simulink model "power_microgrid_v3_analytic"  (R2018b)
settings: Solver=ode23tb  StartTime=0.0  StopTime=24*60*60  FixedStep=1/(1000)  MaxStep=60  RelTol=1e-4
PreLoadFcn:
  | load('solar_load_data_24h.mat')
PostLoadFcn:
  | data = xlsread('Domestic_data_all_x3','Sheet1');
  | breakpoints1 = data(2:end,1)'
  | breakpoints2 = data(1,2:end)
  | table_data = data(2:end,2:end)
undefined symbols (not defined in the file or in its folder): SPD_1min, SPT_1min
libraries: powerlib x24
Description:
  | Copyright 2008-2018 The MathWorks, Inc.
settings Model: ModifiedByFormat=SPS  ExtModeTrigMode=oneshot  ExtModeArmWhenConnect=off  Creator=MathWorks  LastModifiedBy=SPS
settings SolverCC: InitialStep=1e-4  ZeroCrossAlgorithm=Adaptive
settings DataIOCC: SaveFormat=Array  SignalLoggingSaveFormat=ModelDataLogs  SaveOutput=off  SaveTime=off  SignalLoggingName=sigsOut
settings OptimizationCC: BooleanDataType=off  ExpressionDepthLimit=2147483647  InitFltsAndDblsToZero=on  LifeSpan=inf
settings DebuggingCC: AlgebraicLoopMsg=none  SaveWithParameterizedLinksMsg=none  UnderspecifiedInitializationDetection=Classic  MergeDetectMultiDrivingBlocksExec=none  SignalResolutionControl=TryResolveAllWithWarning  MultiTaskDSMMsg=warning  MultiTaskCondExecSysMsg=none  FcnCallInpInsideContextMsg=warning  AllowSymbolicDim=off  StateNameClashWarn=warning  SFUnexpectedBacktrackingDiag=warning  SFNoUnconditionalDefaultTransitionDiag=warning  SFExecutionAtInitializationDiag=none
settings HardwareCC: ProdBitPerPointer=32  ProdBitPerSizeT=32  ProdBitPerPtrDiffT=32  ProdLargestAtomicFloat=None  ProdIntDivRoundTo=Undefined  ProdEndianess=Unspecified  ProdWordSize=32  ProdHWDeviceType=32-bit Generic  TargetUnknown=on
settings ModelReferenceCC: PropagateSignalLabelsOutOfModel=off
settings SFSimCC: SimUseLocalCustomCode=off
settings RTWCC: Description=Generic Real-Time Target  RTWUseLocalCustomCode=off
settings CodeAppCC: StateflowObjectComments=on
settings GRTTargetCC: TargetFcnLib=ansi_tfl_tmw.mat  TargetLangStandard=C89/C90 (ANSI)  GeneratePreprocessorConditionals=Disable all  CombineOutputUpdateFcns=off  GRTInterface=on
settings ConfigComp: CovMetricSettings=dw  CovHtmlReporting=on  CovSaveCumulativeToWorkspaceVar=on  CovSaveSingleToWorkspaceVar=on  CovExternalEMLEnable=off  CovSFcnEnable=off
settings SimscapeCC: SimscapeNormalizeSystem=off

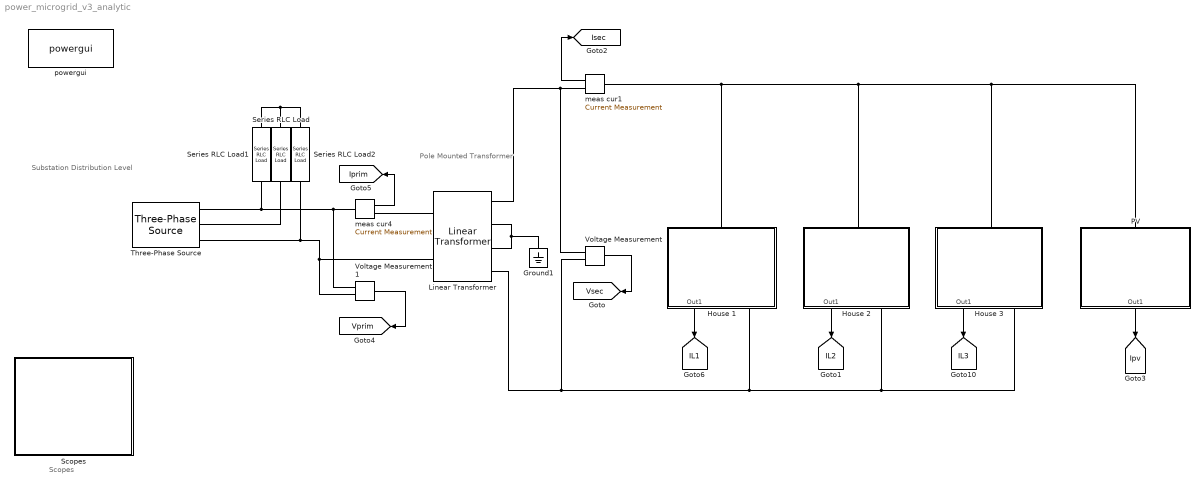
== system power_microgrid_v3_analytic ==
  note: Substation Distribution Level
  note: Pole Mounted
      | Transformer
  note: Scopes
  Ground1 : powerlib/Elements/Ground  LConnTagsString=a
      settings: SourceProductName=Simscape Electrical
  House 1 : Subsystem
      mask Display: image(imread('house.jpg'))
  House 2 : Subsystem
      mask Display: image(imread('house.jpg'))
  House 3 : Subsystem
      mask Display: image(imread('house.jpg'))
  Linear Transformer : powerlib/Elements/Linear Transformer  UNITS=SI  NominalPower=[20e3 50]  winding1=[11e3 0.00005 0.0002]  winding2=[115 0.00005 0.0002]  ThreeWindings=on  winding3=[115 5e-8 2e-8]  RmLm=[50 50]  Measurements=None  DataType=on
      settings: SourceProductName=Simscape Electrical
  PV : Subsystem
      mask Display: image(imread('solar_panel.jpg'))
  Scopes : Subsystem
      mask Display: image(imread('scope.png'))
  Series RLC Load : powerlib/Elements/Series RLC Load  LConnTagsString=a  RConnTagsString=__new0  NominalVoltage=1000  NominalFrequency=50  ActivePower=10e3  InductivePower=100  CapacitivePower=100  Setx0=off  InitialVoltage=0  SetiL0=off  InitialCurrent=0  Measurements=None  LoadType=constant Z
      settings: SourceProductName=Simscape Electrical
  Series RLC Load1 : powerlib/Elements/Series RLC Load  LConnTagsString=a  RConnTagsString=__new0  NominalVoltage=1000  NominalFrequency=50  ActivePower=100e3  InductivePower=100  CapacitivePower=100  Setx0=off  InitialVoltage=0  SetiL0=off  InitialCurrent=0  Measurements=None  LoadType=constant Z
      settings: SourceProductName=Simscape Electrical
  Series RLC Load2 : powerlib/Elements/Series RLC Load  LConnTagsString=a  RConnTagsString=__new0  NominalVoltage=1000  NominalFrequency=50  ActivePower=10e3  InductivePower=100  CapacitivePower=100  Setx0=off  InitialVoltage=0  SetiL0=off  InitialCurrent=0  Measurements=None  LoadType=constant Z
      settings: SourceProductName=Simscape Electrical
  Three-Phase Source : powerlib/Electrical Sources/Three-Phase Source  InternalConnection=Yg  VoltagePhases=off  Voltage=11e3  PhaseAngle=0  Voltage_phases=[25e3 25e3 25e3]/sqrt(3)  PhaseAngles_phases=[0 -120 +120]  Frequency=50  NonIdealSource=off  SpecifyImpedance=on  Resistance=0.8929  Inductance=16.58e-3  ShortCircuitLevel=100e6  BaseVoltage=25e3  XRratio=7  BusType=swing  Pref=0  Qref=0  Prefabc=[10e3, 10e3, 10e3]  Qrefabc=[0, 0, 0]  Qmin=-inf  Qmax=inf
      settings: SourceProductName=Simscape Electrical
  Voltage Measurement : powerlib/Measurements/Voltage Measurement  PhasorSimulation=on  OutputType=Complex  PSBequivalent=0
      settings: SourceProductName=Simscape Electrical
  Voltage Measurement1 : powerlib/Measurements/Voltage Measurement  PhasorSimulation=on  OutputType=Complex  PSBequivalent=0
      settings: SourceProductName=Simscape Electrical
  meas cur1 : powerlib/Measurements/Current Measurement  PhasorSimulation=on  OutputType=Complex  PSBequivalent=0
      settings: SourceProductName=Simscape Electrical
  meas cur4 : powerlib/Measurements/Current Measurement  PhasorSimulation=on  OutputType=Complex  PSBequivalent=0
      settings: SourceProductName=Simscape Electrical
  powergui : powerlib/powergui  SimulationMode=Phasor  SampleTime=1/60/100  frequency=50  Iterations=50  frequencyindice=50  Pbase=100e6  ErrMax=1e-4  UnitsV=kV  UnitsW=MW  buscounter=0  FunctionMessages=off  echomessages=off  EnableUseOfTLC=off  CurrentSourceSwitches=off  DisableSnubberDevices=off  DisableRonSwitches=off  DisableVfSwitches=off  DisplayEquations=off  SolverType=Tustin  Interpol=off  ExternalGateDelay=off  methode=off  Ts=0  x0status=blocks  SPID=off  SwTol=0  HookPort=off  RestoreLinks=warning  ResistiveCurrentMeasurement=off  Frange=[0:2:500]  Ylog=off  Xlog=on  ShowGrid=off  save=off  variable=ZData  structure=0  ZoomFFT=on  StartTime=0.0  cycles=1  DisplayStyle=1  fundamental=60  FreqAxis=off  MaxFrequency=1000  frequencyindicesteady=1  RmsSteady=1  display=off
  tag scope: IL1=global, IL2=global, IL3=global, Iprim=global, Ipv=global, Isec=global, Vprim=global, Vsec=global
  wires:
  House 2/1(Out1) -> [IL2]
  House 1/1(Out1) -> [IL1]
  meas cur1/1 -> [Isec]
  House 3/1(Out1) -> [IL3]
  Voltage Measurement1/1 -> [Vprim]
  meas cur4/1 -> [Iprim]
  Voltage Measurement/1 -> [Vsec]
  PV/1(Out1) -> [Ipv]
  connections:
  Three-Phase Source/RConn1 -- Series RLC Load1/RConn1 -- meas cur4/LConn1 -- Voltage Measurement1/LConn1
  Three-Phase Source/RConn3 -- Series RLC Load2/RConn1 -- Linear Transformer/LConn2 -- Voltage Measurement1/LConn2
  Ground1/LConn1 -- Linear Transformer/RConn2 -- Linear Transformer/RConn3
  Three-Phase Source/RConn2 -- Series RLC Load/RConn1
  Series RLC Load1/LConn1 -- Series RLC Load/LConn1 -- Series RLC Load2/LConn1
  Linear Transformer/LConn1 -- meas cur4/RConn1
  Voltage Measurement/LConn1 -- meas cur1/RConn1 -- Linear Transformer/RConn1
  Voltage Measurement/LConn2 -- House 2/RConn1 -- House 3/RConn1 -- House 1/RConn1 -- Linear Transformer/RConn4
  meas cur1/LConn1 -- PV/LConn1 -- House 3/LConn1 -- House 2/LConn1 -- House 1/LConn1

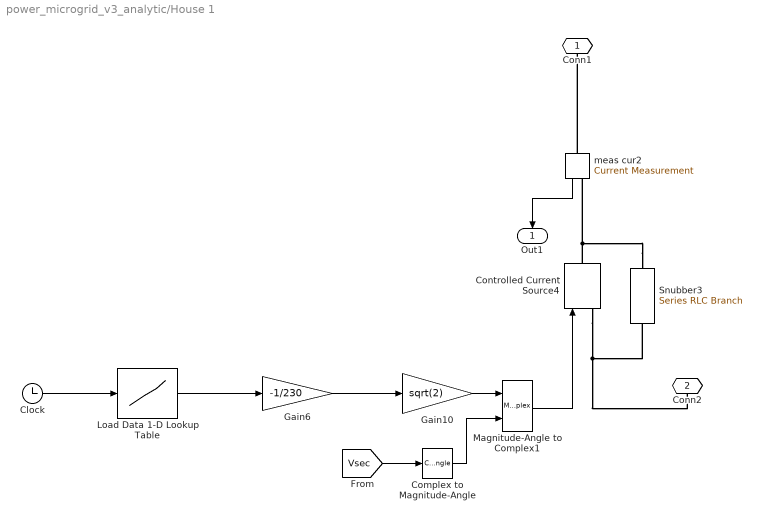
== system power_microgrid_v3_analytic/House 1 ==
  Clock : Clock
  Complex to Magnitude-Angle : ComplexToMagnitudeAngle  Output=Angle
  Controlled Current Source4 : powerlib/Electrical Sources/Controlled Current Source  Initialize=on  Source_Type=AC  Amplitude=0  Phase=0  Frequency=50  Measurements=None
      settings: SourceProductName=Simscape Electrical
  Gain10 : Gain  Gain=sqrt(2)
  Gain6 : Gain  Gain=-1/230
  Load Data 1-D Lookup Table : Lookup_n-D  NumberOfTableDimensions=1  BreakpointsForDimension1="[0.00\t600.00\t1200.00\t1800.00\t2400.00\t3000.00\t3600.00\t4200.00\t4800.00\t5400.00\t6000.00\t6600.00\t7200.00\t7800.00\t8400.00\t9000.00\t9600.00\t10200.00\t10800.00\t11400.00\t12000.00\t12600.00\t13200.00\t13800.00\t14400.00\t15000.00\t15600.00\t16200.00\t16800.00\t17400.00\t18000.00\t18600.00\t19200.00\t19800.00\t20400.00\t21000.00\t21600.00\t22200.00\t22800.00\t23400.00\t24000.00\t24600.00\t25200.00\t25800.00\t26400.00\t27000.00\t27600.00\t28200.00\t28800.00\t29400.00\t30000.00\t30600.00\t31200.00\t31800.00\t32400.00\t33000.00\t33600.00\t34200.00\t34800.00\t35400.00\t36000.00\t36600.00\t37200.00\t37800.00\t38400.00\t39000.00\t39600.00\t40200.00\t40800.00\t41400.00\t42000.00\t42600.00\t43200.00\t43800.00\t44400.00\t45000.00\t45600.00\t46200.00\t46800.00\t47400.00\t48000.00\t48600.00\t49200.00\t49800.00\t50400.00\t51000.00\t51600.00\t52200.00\t52800.00\t53400.00\t54000.00\t54600.00\t55200.00\t55800.00\t56400.00\t57000.00\t57600.00\t58200.00\t58800.00\t59400.00\t60000.00\t60600.00\t61200.00\t61800.00\t62400.00\t63000.00\t63600.00\t64200.00\t64800.00\t65400.00\t66000.00\t66600.00\t67200.00\t67800.00\t68400.00\t69000.00\t69600.00\t70200.00\t70800.00\t71400.00\t72000.00\t72600.00\t73200.00\t73800.00\t74400.00\t75000.00\t75600.00\t76200.00\t76800.00\t77400.00\t78000.00\t78600.00\t79200.00\t79800.00\t80400.00\t81000.00\t81600.00\t82200.00\t82800.00\t83400.00\t84000.00\t84600.00\t85200.00\t85800.00\t86400.00]"  BeginIndexSearchUsingPreviousIndexResult=on  Table="[269.12\t268.66\t262.88\t253.36\t244.82\t234.24\t228.40\t238.53\t239.90\t236.61\t234.08\t222.41\t213.75\t208.20\t197.03\t191.32\t187.67\t187.07\t184.01\t181.34\t180.68\t184.18\t194.62\t200.20\t217.04\t212.93\t205.01\t193.66\t191.08\t179.64\t183.70\t192.56\t191.93\t194.45\t214.76\t219.60\t234.31\t234.64\t258.53\t254.83\t267.04\t284.20\t297.88\t317.55\t332.13\t370.93\t384.15\t384.58\t420.18\t439.42\t431.46\t432.53\t416.15\t423.57\t414.90\t433.96\t442.70\t441.51\t425.40\t424.73\t420.71\t418.26\t419.81\t414.91\t391.96\t387.47\t385.54\t389.59\t407.43\t398.64\t401.19\t404.88\t406.30\t418.06\t411.70\t411.65\t405.44\t393.64\t400.03\t400.28\t393.95\t386.69\t384.67\t381.06\t375.80\t372.99\t371.82\t376.62\t373.59\t367.47\t375.66\t380.24\t391.51\t403.52\t397.48\t406.89\t423.50\t437.56\t449.43\t470.74\t493.19\t510.87\t527.72\t525.40\t532.71\t547.08\t564.42\t582.90\t584.46\t591.07\t577.55\t578.23\t582.92\t579.37\t578.37\t586.69\t583.44\t593.42\t574.46\t580.59\t565.39\t566.30\t555.71\t551.16\t543.74\t532.97\t529.17\t528.60\t520.76\t514.30\t505.98\t493.44\t477.21\t475.17\t463.48\t449.58\t435.67\t410.56\t388.75\t365.41\t346.77\t330.68\t312.41\t291.55\t269.12]"  InternalRulePriority=Speed  RndMeth=Simplest  InputSameDT=on
  Magnitude-Angle to Complex1 : MagnitudeAngleToComplex
  Snubber3 : powerlib/Elements/Series RLC Branch  LConnTagsString=__new0  RConnTagsString=__new0  BranchType=R  Resistance=1e6  Inductance=1e-3  SetiL0=off  InitialCurrent=0  Capacitance=1e-6  Setx0=off  InitialVoltage=0  Measurements=None
      settings: SourceProductName=Simscape Electrical
  meas cur2 : powerlib/Measurements/Current Measurement  PhasorSimulation=on  OutputType=Complex  PSBequivalent=0
      settings: SourceProductName=Simscape Electrical
  Conn1 : PMIOPort  Side=Left
  Conn2 : PMIOPort  Port=2  Side=Right
  Out1 : Outport
  wires:
  Magnitude-Angle to Complex1/1 -> Controlled Current Source4/1
  meas cur2/1 -> Out1/1
  Clock/1 -> Load Data 1-D Lookup Table/1
  Load Data 1-D Lookup Table/1 -> Gain6/1
  [Vsec] -> Complex to Magnitude-Angle/1
  Gain6/1 -> Gain10/1
  Gain10/1 -> Magnitude-Angle to Complex1/1
  Complex to Magnitude-Angle/1 -> Magnitude-Angle to Complex1/2
  connections:
  meas cur2/LConn1 -- Conn1/RConn1
  Snubber3/LConn1 -- Controlled Current Source4/RConn1 -- meas cur2/RConn1
  Snubber3/RConn1 -- Controlled Current Source4/LConn1 -- Conn2/RConn1

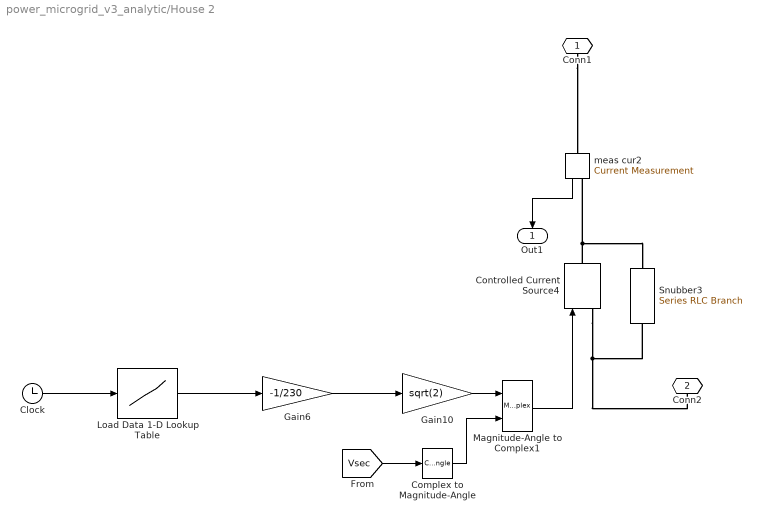
== system power_microgrid_v3_analytic/House 2 ==
  Clock : Clock
  Complex to Magnitude-Angle : ComplexToMagnitudeAngle  Output=Angle
  Controlled Current Source4 : powerlib/Electrical Sources/Controlled Current Source  Initialize=on  Source_Type=AC  Amplitude=0  Phase=0  Frequency=50  Measurements=None
      settings: SourceProductName=Simscape Electrical
  Gain10 : Gain  Gain=sqrt(2)
  Gain6 : Gain  Gain=-1/230
  Load Data 1-D Lookup Table : Lookup_n-D  NumberOfTableDimensions=1  BreakpointsForDimension1="[0.00\t600.00\t1200.00\t1800.00\t2400.00\t3000.00\t3600.00\t4200.00\t4800.00\t5400.00\t6000.00\t6600.00\t7200.00\t7800.00\t8400.00\t9000.00\t9600.00\t10200.00\t10800.00\t11400.00\t12000.00\t12600.00\t13200.00\t13800.00\t14400.00\t15000.00\t15600.00\t16200.00\t16800.00\t17400.00\t18000.00\t18600.00\t19200.00\t19800.00\t20400.00\t21000.00\t21600.00\t22200.00\t22800.00\t23400.00\t24000.00\t24600.00\t25200.00\t25800.00\t26400.00\t27000.00\t27600.00\t28200.00\t28800.00\t29400.00\t30000.00\t30600.00\t31200.00\t31800.00\t32400.00\t33000.00\t33600.00\t34200.00\t34800.00\t35400.00\t36000.00\t36600.00\t37200.00\t37800.00\t38400.00\t39000.00\t39600.00\t40200.00\t40800.00\t41400.00\t42000.00\t42600.00\t43200.00\t43800.00\t44400.00\t45000.00\t45600.00\t46200.00\t46800.00\t47400.00\t48000.00\t48600.00\t49200.00\t49800.00\t50400.00\t51000.00\t51600.00\t52200.00\t52800.00\t53400.00\t54000.00\t54600.00\t55200.00\t55800.00\t56400.00\t57000.00\t57600.00\t58200.00\t58800.00\t59400.00\t60000.00\t60600.00\t61200.00\t61800.00\t62400.00\t63000.00\t63600.00\t64200.00\t64800.00\t65400.00\t66000.00\t66600.00\t67200.00\t67800.00\t68400.00\t69000.00\t69600.00\t70200.00\t70800.00\t71400.00\t72000.00\t72600.00\t73200.00\t73800.00\t74400.00\t75000.00\t75600.00\t76200.00\t76800.00\t77400.00\t78000.00\t78600.00\t79200.00\t79800.00\t80400.00\t81000.00\t81600.00\t82200.00\t82800.00\t83400.00\t84000.00\t84600.00\t85200.00\t85800.00\t86400.00]"  BeginIndexSearchUsingPreviousIndexResult=on  Table="[892.68\t857.87\t634.42\t533.13\t515.24\t533.35\t503.63\t485.43\t489.51\t503.44\t501.81\t494.05\t494.17\t488.46\t494.03\t490.02\t482.00\t502.55\t476.11\t465.11\t410.72\t407.65\t536.82\t467.07\t455.41\t462.20\t441.89\t415.66\t410.61\t436.34\t452.10\t430.78\t389.18\t400.59\t414.76\t385.06\t321.11\t372.36\t344.89\t294.45\t331.14\t313.85\t447.73\t381.69\t385.52\t324.04\t268.08\t353.87\t316.19\t297.07\t236.51\t263.95\t316.11\t296.84\t285.81\t264.30\t283.68\t237.26\t247.29\t273.60\t288.31\t260.70\t255.00\t262.30\t278.30\t341.53\t410.87\t438.85\t381.04\t371.49\t380.51\t357.06\t391.24\t349.66\t372.58\t327.69\t355.61\t525.11\t199.21\t208.77\t250.89\t199.96\t186.56\t203.79\t179.42\t148.99\t156.92\t148.63\t155.69\t178.55\t205.23\t220.36\t209.29\t199.10\t203.84\t185.47\t192.91\t183.40\t194.31\t218.62\t226.20\t252.75\t305.76\t347.19\t396.20\t392.11\t377.60\t320.49\t351.35\t338.95\t345.45\t307.19\t336.80\t340.11\t355.61\t345.44\t342.16\t331.35\t309.51\t283.68\t281.10\t289.12\t279.69\t298.20\t294.80\t307.74\t310.93\t340.29\t364.75\t367.48\t349.98\t417.33\t393.49\t333.47\t342.01\t356.53\t286.11\t282.47\t254.74\t245.94\t227.68\t246.32\t816.12\t926.82\t892.68]"  InternalRulePriority=Speed  RndMeth=Simplest  InputSameDT=on
  Magnitude-Angle to Complex1 : MagnitudeAngleToComplex
  Snubber3 : powerlib/Elements/Series RLC Branch  LConnTagsString=__new0  RConnTagsString=__new0  BranchType=R  Resistance=1e6  Inductance=1e-3  SetiL0=off  InitialCurrent=0  Capacitance=1e-6  Setx0=off  InitialVoltage=0  Measurements=None
      settings: SourceProductName=Simscape Electrical
  meas cur2 : powerlib/Measurements/Current Measurement  PhasorSimulation=on  OutputType=Complex  PSBequivalent=0
      settings: SourceProductName=Simscape Electrical
  Conn1 : PMIOPort  Side=Left
  Conn2 : PMIOPort  Port=2  Side=Right
  Out1 : Outport
  wires:
  meas cur2/1 -> Out1/1
  Clock/1 -> Load Data 1-D Lookup Table/1
  Magnitude-Angle to Complex1/1 -> Controlled Current Source4/1
  Load Data 1-D Lookup Table/1 -> Gain6/1
  Complex to Magnitude-Angle/1 -> Magnitude-Angle to Complex1/2
  Gain10/1 -> Magnitude-Angle to Complex1/1
  Gain6/1 -> Gain10/1
  [Vsec] -> Complex to Magnitude-Angle/1
  connections:
  Controlled Current Source4/LConn1 -- Conn2/RConn1 -- Snubber3/RConn1
  Controlled Current Source4/RConn1 -- meas cur2/RConn1 -- Snubber3/LConn1
  Conn1/RConn1 -- meas cur2/LConn1

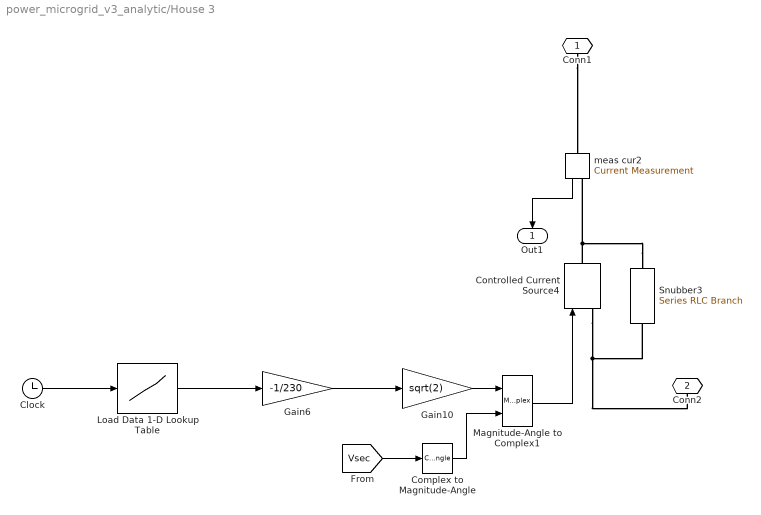
== system power_microgrid_v3_analytic/House 3 ==
  Clock : Clock
  Complex to Magnitude-Angle : ComplexToMagnitudeAngle  Output=Angle
  Controlled Current Source4 : powerlib/Electrical Sources/Controlled Current Source  Initialize=on  Source_Type=AC  Amplitude=0  Phase=0  Frequency=50  Measurements=None
      settings: SourceProductName=Simscape Electrical
  Gain10 : Gain  Gain=sqrt(2)
  Gain6 : Gain  Gain=-1/230
  Load Data 1-D Lookup Table : Lookup_n-D  NumberOfTableDimensions=1  BreakpointsForDimension1="[0.00\t600.00\t1200.00\t1800.00\t2400.00\t3000.00\t3600.00\t4200.00\t4800.00\t5400.00\t6000.00\t6600.00\t7200.00\t7800.00\t8400.00\t9000.00\t9600.00\t10200.00\t10800.00\t11400.00\t12000.00\t12600.00\t13200.00\t13800.00\t14400.00\t15000.00\t15600.00\t16200.00\t16800.00\t17400.00\t18000.00\t18600.00\t19200.00\t19800.00\t20400.00\t21000.00\t21600.00\t22200.00\t22800.00\t23400.00\t24000.00\t24600.00\t25200.00\t25800.00\t26400.00\t27000.00\t27600.00\t28200.00\t28800.00\t29400.00\t30000.00\t30600.00\t31200.00\t31800.00\t32400.00\t33000.00\t33600.00\t34200.00\t34800.00\t35400.00\t36000.00\t36600.00\t37200.00\t37800.00\t38400.00\t39000.00\t39600.00\t40200.00\t40800.00\t41400.00\t42000.00\t42600.00\t43200.00\t43800.00\t44400.00\t45000.00\t45600.00\t46200.00\t46800.00\t47400.00\t48000.00\t48600.00\t49200.00\t49800.00\t50400.00\t51000.00\t51600.00\t52200.00\t52800.00\t53400.00\t54000.00\t54600.00\t55200.00\t55800.00\t56400.00\t57000.00\t57600.00\t58200.00\t58800.00\t59400.00\t60000.00\t60600.00\t61200.00\t61800.00\t62400.00\t63000.00\t63600.00\t64200.00\t64800.00\t65400.00\t66000.00\t66600.00\t67200.00\t67800.00\t68400.00\t69000.00\t69600.00\t70200.00\t70800.00\t71400.00\t72000.00\t72600.00\t73200.00\t73800.00\t74400.00\t75000.00\t75600.00\t76200.00\t76800.00\t77400.00\t78000.00\t78600.00\t79200.00\t79800.00\t80400.00\t81000.00\t81600.00\t82200.00\t82800.00\t83400.00\t84000.00\t84600.00\t85200.00\t85800.00\t86400.00]"  BeginIndexSearchUsingPreviousIndexResult=on  Table="[479.29\t482.54\t450.16\t435.21\t368.89\t333.60\t322.53\t305.93\t301.86\t294.23\t287.52\t274.48\t270.01\t268.26\t256.88\t252.82\t250.51\t254.79\t256.44\t253.44\t250.49\t248.27\t255.22\t278.51\t280.70\t284.79\t269.62\t269.17\t263.40\t253.93\t261.95\t266.81\t273.33\t268.28\t281.22\t292.19\t301.31\t332.72\t319.51\t344.29\t396.35\t473.55\t518.83\t556.59\t579.19\t574.07\t590.21\t629.60\t631.84\t606.56\t638.93\t607.81\t606.55\t607.77\t615.87\t581.32\t574.32\t587.92\t603.57\t585.32\t578.72\t598.86\t584.12\t574.47\t570.88\t579.58\t583.49\t580.46\t587.16\t574.02\t564.59\t569.32\t598.59\t606.11\t595.04\t605.60\t607.79\t603.02\t585.38\t588.59\t581.66\t572.02\t571.23\t567.92\t559.17\t561.94\t547.41\t549.86\t568.38\t581.10\t593.11\t580.91\t589.80\t578.47\t612.90\t620.04\t634.06\t679.98\t693.50\t730.41\t762.44\t771.78\t825.17\t846.48\t853.11\t877.97\t893.34\t911.50\t915.94\t934.64\t923.07\t908.16\t914.35\t908.55\t916.00\t920.77\t883.54\t884.81\t881.02\t892.04\t882.36\t875.27\t871.11\t860.69\t846.93\t847.09\t835.67\t821.60\t787.93\t774.47\t742.58\t727.04\t711.78\t694.40\t662.61\t647.39\t677.79\t667.76\t660.90\t629.36\t587.70\t574.88\t543.50\t520.16\t479.29]"  InternalRulePriority=Speed  RndMeth=Simplest  InputSameDT=on
  Magnitude-Angle to Complex1 : MagnitudeAngleToComplex
  Snubber3 : powerlib/Elements/Series RLC Branch  LConnTagsString=__new0  RConnTagsString=__new0  BranchType=R  Resistance=1e6  Inductance=1e-3  SetiL0=off  InitialCurrent=0  Capacitance=1e-6  Setx0=off  InitialVoltage=0  Measurements=None
      settings: SourceProductName=Simscape Electrical
  meas cur2 : powerlib/Measurements/Current Measurement  PhasorSimulation=on  OutputType=Complex  PSBequivalent=0
      settings: SourceProductName=Simscape Electrical
  Conn1 : PMIOPort  Side=Left
  Conn2 : PMIOPort  Port=2  Side=Right
  Out1 : Outport
  wires:
  meas cur2/1 -> Out1/1
  Clock/1 -> Load Data 1-D Lookup Table/1
  Magnitude-Angle to Complex1/1 -> Controlled Current Source4/1
  Load Data 1-D Lookup Table/1 -> Gain6/1
  Complex to Magnitude-Angle/1 -> Magnitude-Angle to Complex1/2
  Gain10/1 -> Magnitude-Angle to Complex1/1
  Gain6/1 -> Gain10/1
  [Vsec] -> Complex to Magnitude-Angle/1
  connections:
  Conn1/RConn1 -- meas cur2/LConn1
  Snubber3/LConn1 -- meas cur2/RConn1 -- Controlled Current Source4/RConn1
  Snubber3/RConn1 -- Controlled Current Source4/LConn1 -- Conn2/RConn1

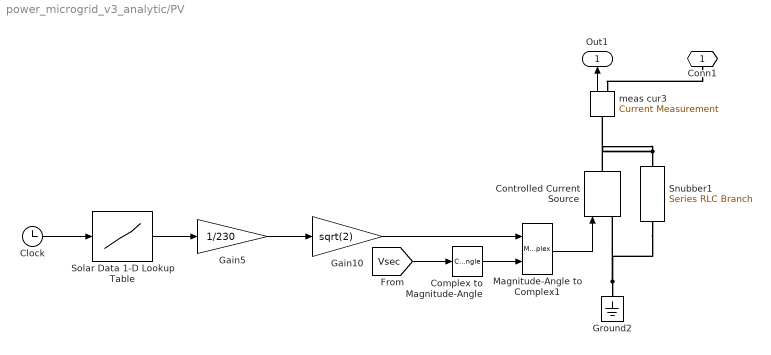
== system power_microgrid_v3_analytic/PV ==
  Clock : Clock
  Complex to Magnitude-Angle : ComplexToMagnitudeAngle  Output=Angle
  Controlled Current Source : powerlib/Electrical Sources/Controlled Current Source  Initialize=on  Source_Type=AC  Amplitude=0  Phase=0  Frequency=50  Measurements=None
      settings: SourceProductName=Simscape Electrical
  Gain10 : Gain  Gain=sqrt(2)
  Gain5 : Gain  Gain=1/230
  Ground2 : powerlib/Elements/Ground  LConnTagsString=a
      settings: SourceProductName=Simscape Electrical
  Magnitude-Angle to Complex1 : MagnitudeAngleToComplex
  Snubber1 : powerlib/Elements/Series RLC Branch  LConnTagsString=__new0  RConnTagsString=__new0  BranchType=R  Resistance=1e6  Inductance=1e-3  SetiL0=off  InitialCurrent=0  Capacitance=1e-6  Setx0=off  InitialVoltage=0  Measurements=None
      settings: SourceProductName=Simscape Electrical
  Solar Data 1-D Lookup Table : Lookup_n-D  NumberOfTableDimensions=1  BreakpointsForDimension1=SPT_1min  BeginIndexSearchUsingPreviousIndexResult=on  Table=SPD_1min  InternalRulePriority=Speed  RndMeth=Simplest  InputSameDT=on
  meas cur3 : powerlib/Measurements/Current Measurement  PhasorSimulation=on  OutputType=Complex  PSBequivalent=0
      settings: SourceProductName=Simscape Electrical
  Conn1 : PMIOPort  Side=Left
  Out1 : Outport
  wires:
  meas cur3/1 -> Out1/1
  Magnitude-Angle to Complex1/1 -> Controlled Current Source/1
  Clock/1 -> Solar Data 1-D Lookup Table/1
  Solar Data 1-D Lookup Table/1 -> Gain5/1
  Gain5/1 -> Gain10/1
  Gain10/1 -> Magnitude-Angle to Complex1/1
  Complex to Magnitude-Angle/1 -> Magnitude-Angle to Complex1/2
  [Vsec] -> Complex to Magnitude-Angle/1
  connections:
  Ground2/LConn1 -- Controlled Current Source/LConn1 -- Snubber1/RConn1
  Snubber1/LConn1 -- Controlled Current Source/RConn1 -- meas cur3/LConn1
  Conn1/RConn1 -- meas cur3/RConn1

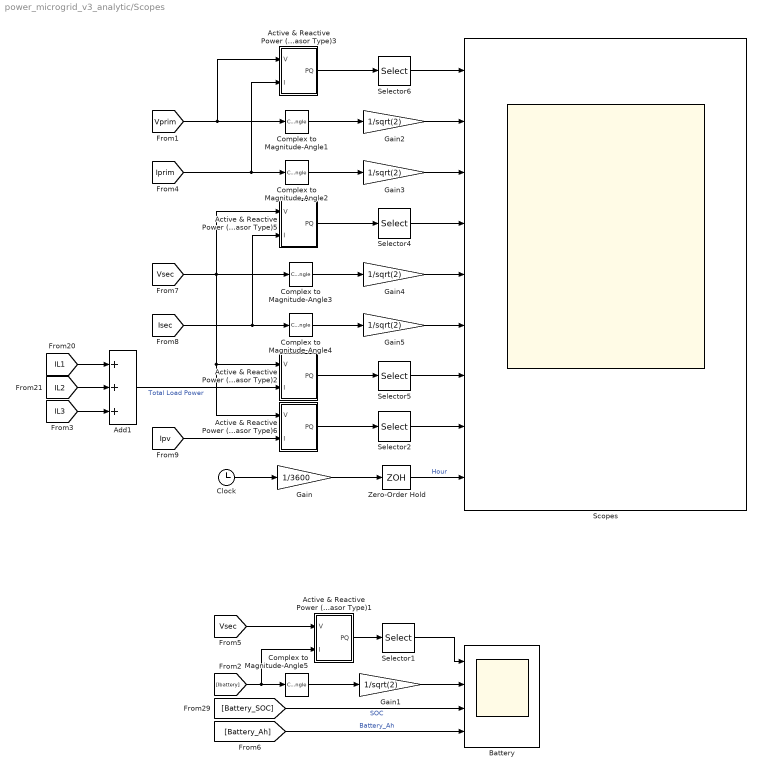
== system power_microgrid_v3_analytic/Scopes ==
  Active & Reactive Power (Phasor Type)1 : Subsystem  DialogController=POWERSYS.PowerSysDialog  mask(Active & Reactive Power (Phasor Type)){}
      mask help: Active & Reactive Power (Phasor Type)
      mask init:
      | power_initmask();
      mask Help: This block is part of a subset of blocks in the Extras library that does not have documentation associated with it, other than the block mask description.
      mask Display: disp('')
  Active & Reactive Power (Phasor Type)2 : Subsystem  DialogController=POWERSYS.PowerSysDialog  mask(Active & Reactive Power (Phasor Type)){}
      mask help: Active & Reactive Power (Phasor Type)
      mask init:
      | power_initmask();
      mask Help: This block is part of a subset of blocks in the Extras library that does not have documentation associated with it, other than the block mask description.
      mask Display: disp('')
  Active & Reactive Power (Phasor Type)3 : Subsystem  DialogController=POWERSYS.PowerSysDialog  mask(Active & Reactive Power (Phasor Type)){}
      mask help: Active & Reactive Power (Phasor Type)
      mask init:
      | power_initmask();
      mask Help: This block is part of a subset of blocks in the Extras library that does not have documentation associated with it, other than the block mask description.
      mask Display: disp('')
  Active & Reactive Power (Phasor Type)5 : Subsystem  DialogController=POWERSYS.PowerSysDialog  mask(Active & Reactive Power (Phasor Type)){}
      mask help: Active & Reactive Power (Phasor Type)
      mask init:
      | power_initmask();
      mask Help: This block is part of a subset of blocks in the Extras library that does not have documentation associated with it, other than the block mask description.
      mask Display: disp('')
  Active & Reactive Power (Phasor Type)6 : Subsystem  DialogController=POWERSYS.PowerSysDialog  mask(Active & Reactive Power (Phasor Type)){}
      mask help: Active & Reactive Power (Phasor Type)
      mask init:
      | power_initmask();
      mask Help: This block is part of a subset of blocks in the Extras library that does not have documentation associated with it, other than the block mask description.
      mask Display: disp('')
  Add1 : Sum  Inputs=+++
  Battery : Scope  NumInputPorts=4
  Clock : Clock
  Complex to Magnitude-Angle{1..5} (5 alike) : ComplexToMagnitudeAngle  Output=Magnitude
  Gain : Gain  Gain=1/3600
  Gain{1..5} (5 alike) : Gain  Gain=1/sqrt(2)
  Scopes : Scope  NumInputPorts=9
  Selector{1..2,4..6} (5 alike) : Selector  InputPortWidth=2  IndexOptions=Index vector (dialog)  Indices=1  OutputSizes=1
  Zero-Order Hold : ZeroOrderHold  SampleTime=3600
  wires:
  Clock/1 -> Gain/1
  Gain/1 -> Zero-Order Hold/1
  Zero-Order Hold/1 -> Scopes/9  "Hour"
  Gain2/1 -> Scopes/2
  [Vprim] -> Complex to Magnitude-Angle1/1, Active & Reactive Power (Phasor Type)3/1(V)
  [Iprim] -> Complex to Magnitude-Angle2/1, Active & Reactive Power (Phasor Type)3/2(I)
  Gain3/1 -> Scopes/3
  [Vsec] -> Complex to Magnitude-Angle3/1, Active & Reactive Power (Phasor Type)6/1(V), Active & Reactive Power (Phasor Type)2/1(V), Active & Reactive Power (Phasor Type)5/1(V)
  Gain4/1 -> Scopes/5
  [Isec] -> Complex to Magnitude-Angle4/1, Active & Reactive Power (Phasor Type)5/2(I)
  Gain5/1 -> Scopes/6
  Selector6/1 -> Scopes/1
  Active & Reactive Power (Phasor Type)3/1(PQ) -> Selector6/1
  Selector4/1 -> Scopes/4
  Active & Reactive Power (Phasor Type)5/1(PQ) -> Selector4/1
  [IL2] -> Add1/2
  [IL1] -> Add1/1
  [IL3] -> Add1/3
  Active & Reactive Power (Phasor Type)2/1(PQ) -> Selector5/1
  Selector5/1 -> Scopes/7
  Add1/1 -> Active & Reactive Power (Phasor Type)2/2(I)  "Total Load Power"
  [Ipv] -> Active & Reactive Power (Phasor Type)6/2(I)
  Active & Reactive Power (Phasor Type)6/1(PQ) -> Selector2/1
  Selector2/1 -> Scopes/8
  [Battery_Ah] -> Battery/4  "Battery_Ah"
  [Battery_SOC] -> Battery/3  "SOC"
  [Ibattery] -> Active & Reactive Power (Phasor Type)1/2(I), Complex to Magnitude-Angle5/1
  Complex to Magnitude-Angle5/1 -> Gain1/1
  Gain1/1 -> Battery/2
  Active & Reactive Power (Phasor Type)1/1(PQ) -> Selector1/1
  Selector1/1 -> Battery/1
  [Vsec] -> Active & Reactive Power (Phasor Type)1/1(V)
  Complex to Magnitude-Angle1/1 -> Gain2/1
  Complex to Magnitude-Angle2/1 -> Gain3/1
  Complex to Magnitude-Angle3/1 -> Gain4/1
  Complex to Magnitude-Angle4/1 -> Gain5/1

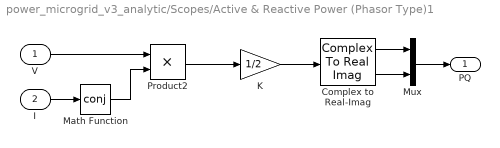
== system power_microgrid_v3_analytic/Scopes/Active & Reactive Power (Phasor Type)1 ==
  V : Inport
  I : Inport  Port=2
  Complex to Real-Imag : ComplexToRealImag
  K : Gain  Gain=1/2  SaturateOnIntegerOverflow=on  OutDataTypeStr=Inherit: Same as input  ParamDataTypeStr=Inherit: Same as input
  Math Function : Math  Operator=conj  SaturateOnIntegerOverflow=on
  Mux : Mux  Inputs=2
  Product2 : Product  SaturateOnIntegerOverflow=on  InputSameDT=on  OutDataTypeStr=Inherit: Same as first input
  PQ : Outport
  wires:
  Mux/1 -> PQ/1
  Complex to Real-Imag/2 -> Mux/2
  Complex to Real-Imag/1 -> Mux/1
  V/1 -> Product2/1
  Math Function/1 -> Product2/2
  Product2/1 -> K/1
  K/1 -> Complex to Real-Imag/1
  I/1 -> Math Function/1

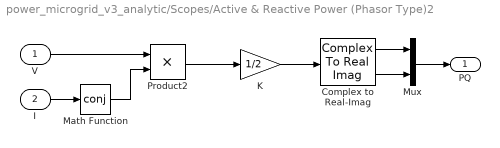
== system power_microgrid_v3_analytic/Scopes/Active & Reactive Power (Phasor Type)2 ==
  V : Inport
  I : Inport  Port=2
  Complex to Real-Imag : ComplexToRealImag
  K : Gain  Gain=1/2  SaturateOnIntegerOverflow=on  OutDataTypeStr=Inherit: Same as input  ParamDataTypeStr=Inherit: Same as input
  Math Function : Math  Operator=conj  SaturateOnIntegerOverflow=on
  Mux : Mux  Inputs=2
  Product2 : Product  SaturateOnIntegerOverflow=on  InputSameDT=on  OutDataTypeStr=Inherit: Same as first input
  PQ : Outport
  wires:
  Mux/1 -> PQ/1
  Complex to Real-Imag/2 -> Mux/2
  Complex to Real-Imag/1 -> Mux/1
  V/1 -> Product2/1
  Math Function/1 -> Product2/2
  Product2/1 -> K/1
  K/1 -> Complex to Real-Imag/1
  I/1 -> Math Function/1

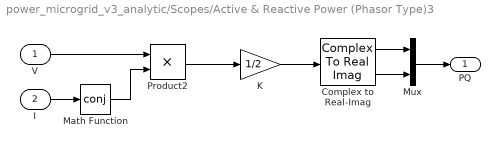
== system power_microgrid_v3_analytic/Scopes/Active & Reactive Power (Phasor Type)3 ==
  V : Inport
  I : Inport  Port=2
  Complex to Real-Imag : ComplexToRealImag
  K : Gain  Gain=1/2  SaturateOnIntegerOverflow=on  OutDataTypeStr=Inherit: Same as input  ParamDataTypeStr=Inherit: Same as input
  Math Function : Math  Operator=conj  SaturateOnIntegerOverflow=on
  Mux : Mux  Inputs=2
  Product2 : Product  SaturateOnIntegerOverflow=on  InputSameDT=on  OutDataTypeStr=Inherit: Same as first input
  PQ : Outport
  wires:
  Mux/1 -> PQ/1
  Complex to Real-Imag/2 -> Mux/2
  Complex to Real-Imag/1 -> Mux/1
  V/1 -> Product2/1
  Math Function/1 -> Product2/2
  Product2/1 -> K/1
  K/1 -> Complex to Real-Imag/1
  I/1 -> Math Function/1

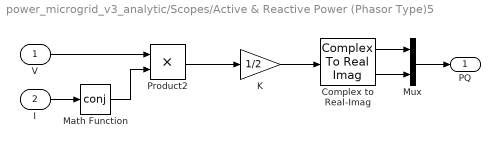
== system power_microgrid_v3_analytic/Scopes/Active & Reactive Power (Phasor Type)5 ==
  V : Inport
  I : Inport  Port=2
  Complex to Real-Imag : ComplexToRealImag
  K : Gain  Gain=1/2  SaturateOnIntegerOverflow=on  OutDataTypeStr=Inherit: Same as input  ParamDataTypeStr=Inherit: Same as input
  Math Function : Math  Operator=conj  SaturateOnIntegerOverflow=on
  Mux : Mux  Inputs=2
  Product2 : Product  SaturateOnIntegerOverflow=on  InputSameDT=on  OutDataTypeStr=Inherit: Same as first input
  PQ : Outport
  wires:
  Mux/1 -> PQ/1
  Complex to Real-Imag/2 -> Mux/2
  Complex to Real-Imag/1 -> Mux/1
  V/1 -> Product2/1
  Math Function/1 -> Product2/2
  Product2/1 -> K/1
  K/1 -> Complex to Real-Imag/1
  I/1 -> Math Function/1

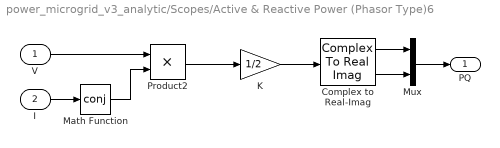
== system power_microgrid_v3_analytic/Scopes/Active & Reactive Power (Phasor Type)6 ==
  V : Inport
  I : Inport  Port=2
  Complex to Real-Imag : ComplexToRealImag
  K : Gain  Gain=1/2  SaturateOnIntegerOverflow=on  OutDataTypeStr=Inherit: Same as input  ParamDataTypeStr=Inherit: Same as input
  Math Function : Math  Operator=conj  SaturateOnIntegerOverflow=on
  Mux : Mux  Inputs=2
  Product2 : Product  SaturateOnIntegerOverflow=on  InputSameDT=on  OutDataTypeStr=Inherit: Same as first input
  PQ : Outport
  wires:
  Mux/1 -> PQ/1
  Complex to Real-Imag/2 -> Mux/2
  Complex to Real-Imag/1 -> Mux/1
  V/1 -> Product2/1
  Math Function/1 -> Product2/2
  Product2/1 -> K/1
  K/1 -> Complex to Real-Imag/1
  I/1 -> Math Function/1
